simulink model "observador_simulink"  (R2024b)
settings: Solver=VariableStepAuto  StartTime=0.0  StopTime=10.0  RelTol=1e-3
values from neighbouring files (symbols this model uses):
  G = eye(2) + A*FI    [servosistema.m]
  H = FI*B    [servosistema.m]
  K1 = -KN(3)    [servosistema.m]
  K2 = KN(1:2)    [servosistema.m]
  Ke = acker(G', C', [zo1 zo2])'    [servosistema.m]
  T = 0.25    [servosistema.m]
settings Model: Creator=syaba  LastModifiedBy=syaba

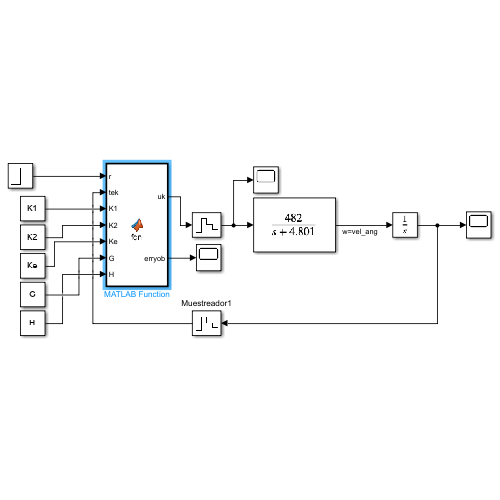
[thumbnail: Simulink's stored preview of the top-level diagram]
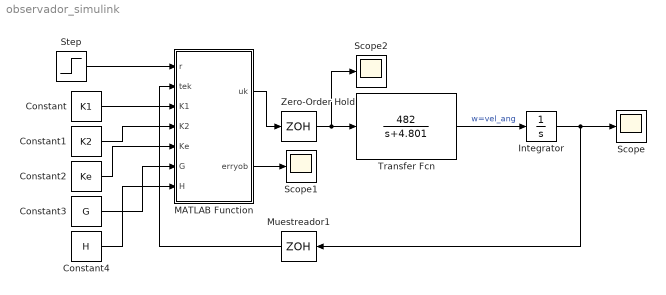
== system observador_simulink ==
  Constant : Constant  Value=K1
  Constant1 : Constant  Value=K2  VectorParams1D=off
  Constant2 : Constant  Value=Ke  VectorParams1D=off
  Constant3 : Constant  Value=G  VectorParams1D=off
  Constant4 : Constant  Value=H  VectorParams1D=off
  Integrator : Integrator
  MATLAB Function : MATLAB Function  TreatAsAtomicUnit=on  SystemSampleTime=T
  Muestreador1 : ZeroOrderHold  SampleTime=T
  Scope : Scope
  Scope1 : Scope
  Scope2 : Scope
  Step : Step  Time=0  After=100  SampleTime=0
  Transfer Fcn : TransferFcn  Numerator=[482]  Denominator=[1 4.801]
  Zero-Order Hold : ZeroOrderHold  SampleTime=T
  wires:
  Transfer Fcn/1 -> Integrator/1  "w=vel_ang"
  MATLAB Function/1(uk) -> Zero-Order Hold/1
  Integrator/1 -> Muestreador1/1, Scope/1
  Constant/1 -> MATLAB Function/3(K1)
  Constant1/1 -> MATLAB Function/4(K2)
  Step/1 -> MATLAB Function/1(r)
  Muestreador1/1 -> MATLAB Function/2(tek)
  Constant2/1 -> MATLAB Function/5(Ke)
  Constant3/1 -> MATLAB Function/6(G)
  Constant4/1 -> MATLAB Function/7(H)
  MATLAB Function/2(erryob) -> Scope1/1
  Zero-Order Hold/1 -> Scope2/1, Transfer Fcn/1

== matlab function observador_simulink/MATLAB Function ==
  data: r input; uk output; tek input; K1 input; K2 input; Ke input; G input; H input; erryob output
function [uk, erryob] = fcn(r, tek, K1, K2, Ke, G, H)

persistent vk_1;
persistent xob;

if isempty(vk_1)
    vk_1 = 0;
    xob = [0;0];
end;

C = [1 0];
ek = r-tek;
vk = vk_1 + ek;
uk = K1*vk - K2*xob;

% xob_m = xob(k+1)
% xob = xob(k)

xob_m = G*xob + H*uk + Ke*(tek-C*xob)
erryob = tek - C*xob;

vk_1 = vk;
xob = xob_m;
